simulink model "ADC"  (Simulink 8.5)
settings: Solver=ode23tb  StartTime=0.0  StopTime=0.25  MaxStep=1e-5  RelTol=1e-9
settings Model: Creator=Shailesh  LastModifiedBy=tesla
settings SolverCC: MaxConsecutiveMinStep=20
settings OptimizationCC: InitFltsAndDblsToZero=on
settings DebuggingCC: SaveWithParameterizedLinksMsg=none  SignalResolutionControl=TryResolveAllWithWarning  SolverPrmCheckMsg=warning  MultiTaskDSMMsg=warning  MultiTaskCondExecSysMsg=none  FcnCallInpInsideContextMsg=UseLocalSettings
settings GRTTargetCC: TargetFcnLib=ansi_tfl_tmw.mat
settings ConfigurationSet: Description=SimMechanics 2G

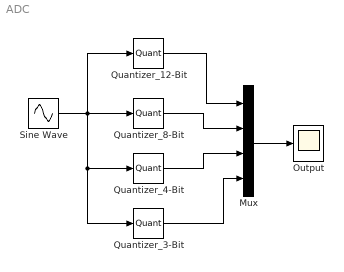
== system ADC ==
  Mux : Mux
  Output : Scope
      settings: YMin=10  YMax=16  MaxDataPoints=5000000
  Quantizer_12-Bit : Quantizer  QuantizationInterval=5/4095
  Quantizer_3-Bit : Quantizer  QuantizationInterval=5/8
  Quantizer_4-Bit : Quantizer  QuantizationInterval=5/15
  Quantizer_8-Bit : Quantizer  QuantizationInterval=5/255
  Sine Wave : Sin  Amplitude=2.5  Frequency=377  SampleTime=0
  wires:
  Sine Wave/1 -> Quantizer_3-Bit/1, Quantizer_4-Bit/1, Quantizer_12-Bit/1, Quantizer_8-Bit/1
  Quantizer_12-Bit/1 -> Mux/1
  Quantizer_8-Bit/1 -> Mux/2
  Quantizer_4-Bit/1 -> Mux/3
  Mux/1 -> Output/1
  Quantizer_3-Bit/1 -> Mux/4
